simulink model "Assignment4Sim"  (R2020b)
settings: Solver=VariableStepAuto  StartTime=0.0  StopTime=20  RelTol=1e-3
values from neighbouring files (symbols this model uses):
  a = 1    [Assignment4Mat.m]
  am = 1    [Assignment4Mat.m]
  amp1 = 1/10    (= 0.1)    [Assignment4Mat.m]
  amp2 = 10    [Assignment4Mat.m]
  ampD = 0.1    [Assignment4Mat.m]
  freq1 = 10    [Assignment4Mat.m]
  freq2 = 1/10    (= 0.1)    [Assignment4Mat.m]
  freqD = 1/5    (= 0.2)    [Assignment4Mat.m]
  gammaMRAC = 1    [Assignment4Mat.m]
  x0 = 1    [Assignment4Mat.m]
settings Model: Creator=Paolo  LastModifiedBy=Paolo

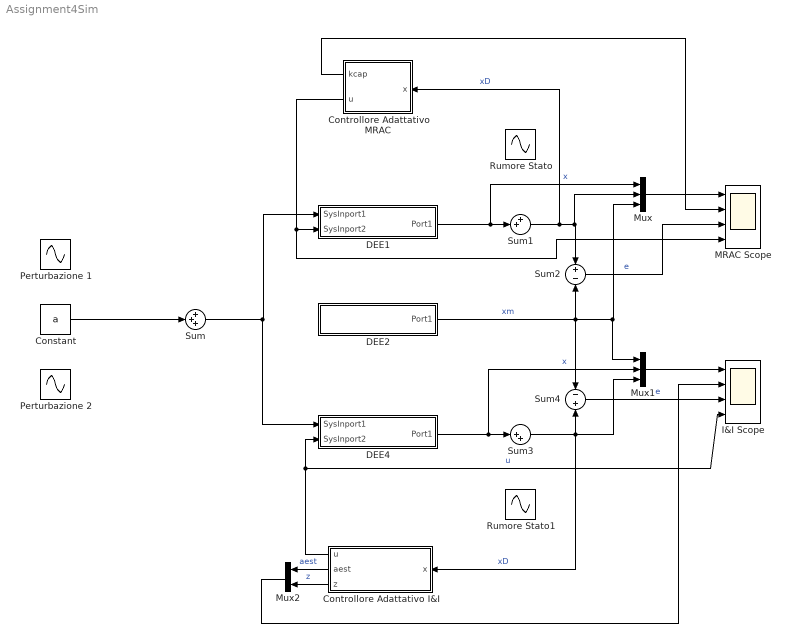
== system Assignment4Sim ==
  "  DEE2 " : Subsystem  mask(Differential Equation Editor (DEE)){}
      settings: OpenFcn=diffeqed
      mask Display: disp('Reference Model')
  Constant : Constant  Value=a
  Controllore Adattativo I&I : Subsystem
  Controllore Adattativo MRAC : Subsystem
  "DEE1 " : Subsystem  mask(Differential Equation Editor (DEE)){}
      settings: OpenFcn=diffeqed
      mask Display: disp('Sistema')
  "DEE4 " : Subsystem  mask(Differential Equation Editor (DEE)){}
      settings: OpenFcn=diffeqed
      mask Display: disp('Sistema')
  I&I Scope : Scope  NumInputPorts=4
  MRAC Scope : Scope  NumInputPorts=4
  Mux : Mux  Inputs=3
  Mux1 : Mux  Inputs=3
  Mux2 : Mux  Inputs=2
  Perturbazione 1 : Sin  Amplitude=amp1  Frequency=freq1  SampleTime=0
  Perturbazione 2 : Sin  Amplitude=amp2  Frequency=freq2  SampleTime=0
  Rumore Stato : Sin  Amplitude=ampD  Frequency=freqD  SampleTime=0
  Rumore Stato1 : Sin  Amplitude=ampD  Frequency=freqD  SampleTime=0
  Sum : Sum  Inputs=+++
  Sum1 : Sum  Inputs=++|
  Sum2 : Sum  Inputs=+|-
  Sum3 : Sum  Inputs=|++
  Sum4 : Sum  Inputs=-|+
  wires:
  Constant/1 -> Sum/2
  Sum/1 -> "DEE4 "/1(SysInport1), "DEE1 "/1(SysInport1)
  "  DEE2 "/1(Port1) -> Sum4/1, Mux1/1, Mux/3, Sum2/2  "xm"
  "DEE1 "/1(Port1) -> Mux/1, Sum1/2  "x"
  Sum1/1 -> Mux/2, Sum2/1, Controllore Adattativo MRAC/1(x)  "xD"
  Controllore Adattativo MRAC/2(u) -> MRAC Scope/4, "DEE1 "/2(SysInport2)
  Sum2/1 -> MRAC Scope/3  "e"
  Mux/1 -> MRAC Scope/1
  Controllore Adattativo MRAC/1(kcap) -> MRAC Scope/2
  "DEE4 "/1(Port1) -> Mux1/2, Sum3/1  "x"
  Sum3/1 -> Controllore Adattativo I&I/1(x), Mux1/3, Sum4/2  "xD"
  Mux1/1 -> I&I Scope/1
  Sum4/1 -> I&I Scope/3  "e"
  Controllore Adattativo I&I/1(u) -> I&I Scope/4, "DEE4 "/2(SysInport2)  "u"
  Controllore Adattativo I&I/2(aest) -> Mux2/1  "aest"
  Controllore Adattativo I&I/3(z) -> Mux2/2  "z"
  Mux2/1 -> I&I Scope/2

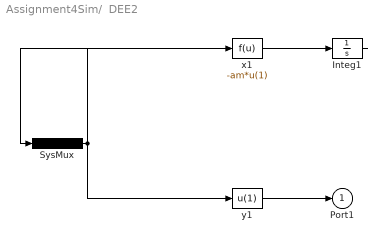
== system Assignment4Sim/  DEE2  ==
  Integ1 : Integrator  InitialCondition=1
  SysMux : Mux  Inputs=1
  x1 : Fcn  Expr=-am*u(1)
  y1 : Fcn  Expr=u(1)
  Port1 : Outport
  wires:
  SysMux/1 -> x1/1, y1/1
  x1/1 -> Integ1/1
  Integ1/1 -> SysMux/1
  y1/1 -> Port1/1

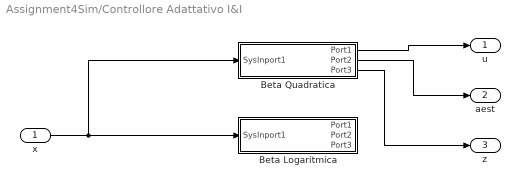
== system Assignment4Sim/Controllore Adattativo I&I ==
  x : Inport
  Beta Logaritmica : Subsystem  mask(Differential Equation Editor (DEE)){}
      settings: OpenFcn=diffeqed
      mask Display: disp('Osservatore I&I 2')
  Beta Quadratica : Subsystem  mask(Differential Equation Editor (DEE)){}
      settings: OpenFcn=diffeqed
      mask Display: disp('Osservatore I&I 1')
  u : Outport
  aest : Outport  Port=2
  z : Outport  Port=3
  wires:
  x/1 -> Beta Logaritmica/1(SysInport1), Beta Quadratica/1(SysInport1)
  Beta Quadratica/1(Port1) -> u/1
  Beta Quadratica/2(Port2) -> aest/1
  Beta Quadratica/3(Port3) -> z/1

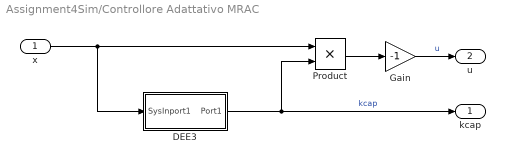
== system Assignment4Sim/Controllore Adattativo MRAC ==
  x : Inport
  " DEE3   " : Subsystem  mask(Differential Equation Editor (DEE)){}
      settings: OpenFcn=diffeqed
      mask Display: disp('Stimatore')
  Gain : Gain  Gain=-1
  Product : Product
  kcap : Outport
  u : Outport  Port=2
  wires:
  Product/1 -> Gain/1
  x/1 -> Product/1, " DEE3   "/1(SysInport1)
  " DEE3   "/1(Port1) -> kcap/1, Product/2  "kcap"
  Gain/1 -> u/1  "u"

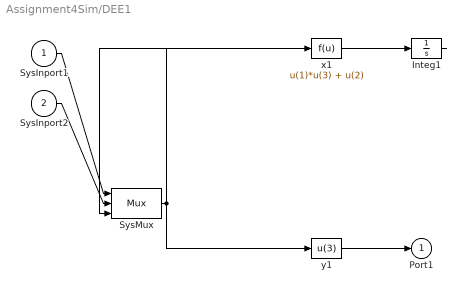
== system Assignment4Sim/DEE1  ==
  SysInport1 : Inport
  SysInport2 : Inport  Port=2
  Integ1 : Integrator  InitialCondition=x0
  SysMux : Mux  Inputs=3
  x1 : Fcn  Expr=u(1)*u(3) + u(2)
  y1 : Fcn  Expr=u(3)
  Port1 : Outport
  wires:
  SysInport1/1 -> SysMux/1
  SysInport2/1 -> SysMux/2
  SysMux/1 -> x1/1, y1/1
  x1/1 -> Integ1/1
  Integ1/1 -> SysMux/3
  y1/1 -> Port1/1

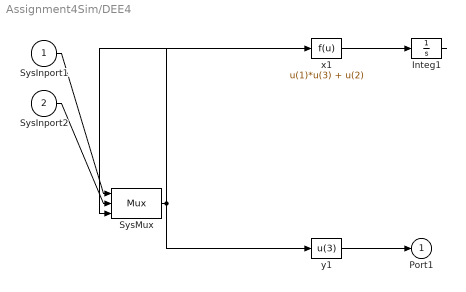
== system Assignment4Sim/DEE4  ==
  SysInport1 : Inport
  SysInport2 : Inport  Port=2
  Integ1 : Integrator  InitialCondition=x0
  SysMux : Mux  Inputs=3
  x1 : Fcn  Expr=u(1)*u(3) + u(2)
  y1 : Fcn  Expr=u(3)
  Port1 : Outport
  wires:
  SysInport1/1 -> SysMux/1
  SysInport2/1 -> SysMux/2
  SysMux/1 -> x1/1, y1/1
  x1/1 -> Integ1/1
  Integ1/1 -> SysMux/3
  y1/1 -> Port1/1

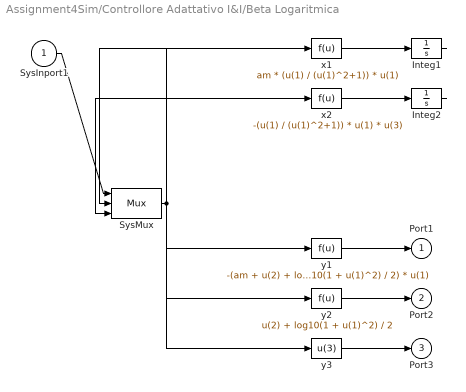
== system Assignment4Sim/Controllore Adattativo I&I/Beta Logaritmica ==
  SysInport1 : Inport
  Integ1 : Integrator
  Integ2 : Integrator  InitialCondition=1
  SysMux : Mux  Inputs=3
  x1 : Fcn  Expr=am * (u(1) / (u(1)^2+1)) * u(1)
  x2 : Fcn  Expr=-(u(1) / (u(1)^2+1)) * u(1) * u(3)
  y1 : Fcn  Expr=-(am + u(2) + log10(1 + u(1)^2) / 2) * u(1)
  y2 : Fcn  Expr=u(2) + log10(1 + u(1)^2) / 2
  y3 : Fcn  Expr=u(3)
  Port1 : Outport
  Port2 : Outport  Port=2
  Port3 : Outport  Port=3
  wires:
  SysInport1/1 -> SysMux/1
  SysMux/1 -> x1/1, x2/1, y1/1, y2/1, y3/1
  x1/1 -> Integ1/1
  Integ1/1 -> SysMux/2
  x2/1 -> Integ2/1
  Integ2/1 -> SysMux/3
  y1/1 -> Port1/1
  y2/1 -> Port2/1
  y3/1 -> Port3/1

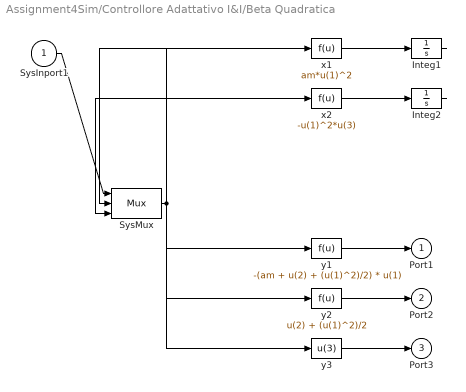
== system Assignment4Sim/Controllore Adattativo I&I/Beta Quadratica ==
  SysInport1 : Inport
  Integ1 : Integrator
  Integ2 : Integrator  InitialCondition=1
  SysMux : Mux  Inputs=3
  x1 : Fcn  Expr=am*u(1)^2
  x2 : Fcn  Expr=-u(1)^2*u(3)
  y1 : Fcn  Expr=-(am + u(2) + (u(1)^2)/2) * u(1)
  y2 : Fcn  Expr=u(2) + (u(1)^2)/2
  y3 : Fcn  Expr=u(3)
  Port1 : Outport
  Port2 : Outport  Port=2
  Port3 : Outport  Port=3
  wires:
  SysInport1/1 -> SysMux/1
  SysMux/1 -> x1/1, x2/1, y1/1, y2/1, y3/1
  x1/1 -> Integ1/1
  Integ1/1 -> SysMux/2
  x2/1 -> Integ2/1
  Integ2/1 -> SysMux/3
  y1/1 -> Port1/1
  y2/1 -> Port2/1
  y3/1 -> Port3/1

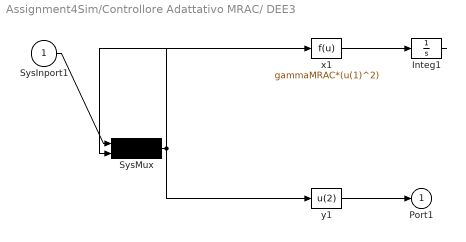
== system Assignment4Sim/Controllore Adattativo MRAC/ DEE3    ==
  SysInport1 : Inport
  Integ1 : Integrator
  SysMux : Mux  Inputs=2
  x1 : Fcn  Expr=gammaMRAC*(u(1)^2)
  y1 : Fcn  Expr=u(2)
  Port1 : Outport
  wires:
  SysInport1/1 -> SysMux/1
  SysMux/1 -> x1/1, y1/1
  x1/1 -> Integ1/1
  Integ1/1 -> SysMux/2
  y1/1 -> Port1/1
